simulink model "AngleSpeedToPWM"  (R2014a)
settings: Solver=FixedStepDiscrete  StartTime=0.0  StopTime=500000  FixedStep=1  RelTol=1e-3
libraries: hdlsllib x3
settings Model: Creator=sun.yifa  LastModifiedBy=rogers.a
settings OptimizationCC: BlockReduction=off  ConditionallyExecuteInputs=off  InlineParams=on
settings DebuggingCC: AlgebraicLoopMsg=error
settings HardwareCC: ProdHWDeviceType=ASIC/FPGA->ASIC/FPGA  ProdEqTarget=off

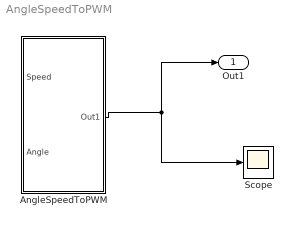
== system AngleSpeedToPWM ==
  "AngleSpeedToPWM " : Subsystem
  Scope : Scope
      settings: SaveName=ScopeData2
  Out1 : Outport  OutDataTypeStr=boolean
  wires:
  "AngleSpeedToPWM "/1(Out1) -> Scope/1, Out1/1

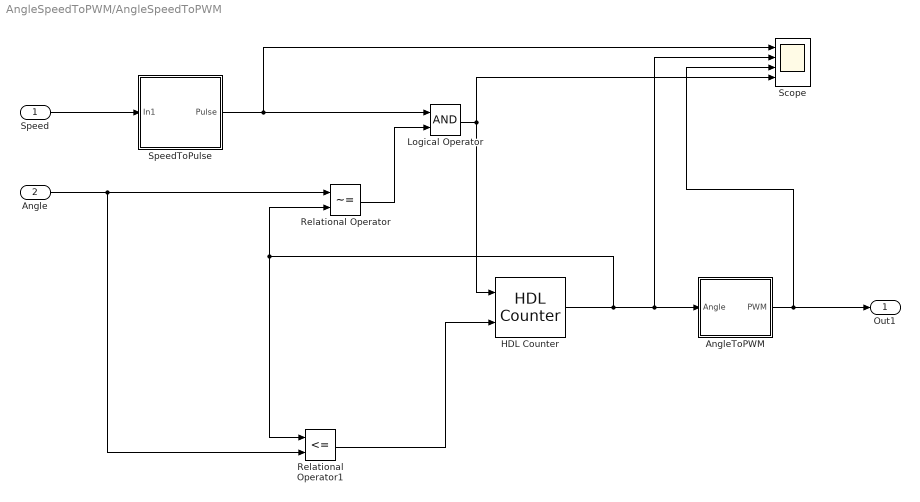
== system AngleSpeedToPWM/AngleSpeedToPWM  ==
  Speed : Inport
  Angle : Inport  Port=2
  "AngleToPWM " : Subsystem
  HDL Counter : hdlsllib/HDL Operations/HDL Counter  CountType=Count limited  CountInit=0  CountStep=1  CountMax=180  CountFromType=Specify  CountFrom=0  CountResetPort=off  CountLoadPort=off  CountEnbPort=on  CountDirPort=on  CountDataType=Unsigned  CountWordLen=8  CountFracLen=0  CountSampTime=1
  Logical Operator : Logic  AllPortsSameDT=off  OutDataTypeStr=boolean
  Relational Operator : RelationalOperator  Operator=~=  OutDataTypeStr=boolean
  Relational Operator1 : RelationalOperator  Operator=<=  OutDataTypeStr=boolean
  Scope : Scope  NumInputPorts=4
      settings: YMin=0~0~0~0  YMax=1~300~1~1
  SpeedToPulse : Subsystem
  Out1 : Outport  OutDataTypeStr=boolean
  wires:
  Speed/1 -> SpeedToPulse/1(In1)
  SpeedToPulse/1(Pulse) -> Logical Operator/1, Scope/1
  Angle/1 -> Relational Operator1/2, Relational Operator/1
  Relational Operator/1 -> Logical Operator/2
  Logical Operator/1 -> HDL Counter/1, Scope/4
  Relational Operator1/1 -> HDL Counter/2
  HDL Counter/1 -> Relational Operator/2, Relational Operator1/1, Scope/2, "AngleToPWM "/1("Angle ")
  "AngleToPWM "/1("PWM ") -> Out1/1, Scope/3

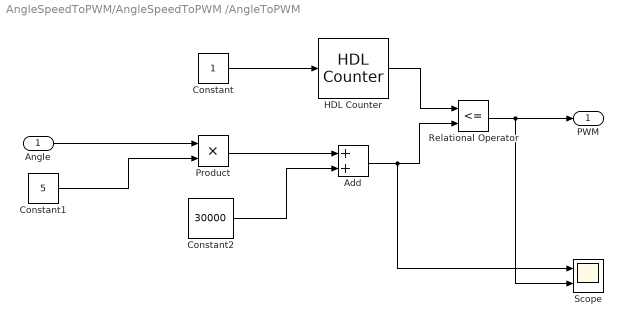
== system AngleSpeedToPWM/AngleSpeedToPWM /AngleToPWM  ==
  "Angle " : Inport  OutDataTypeStr=uint8
  Add : Sum
  Constant : Constant  OutDataTypeStr=boolean
  Constant1 : Constant  Value=5  OutDataTypeStr=uint32
  Constant2 : Constant  Value=30000  OutDataTypeStr=uint32
  HDL Counter : hdlsllib/HDL Operations/HDL Counter  CountType=Count limited  CountInit=0  CountStep=1  CountMax=10000  CountFromType=Initial value  CountFrom=0  CountResetPort=off  CountLoadPort=off  CountEnbPort=on  CountDirPort=off  CountDataType=Unsigned  CountWordLen=32  CountFracLen=0  CountSampTime=1
  Product : Product  OutDataTypeStr=Inherit: Inherit via back propagation  SaturateOnIntegerOverflow=on
  Relational Operator : RelationalOperator  Operator=<=  OutDataTypeStr=boolean
  Scope : Scope  NumInputPorts=2
      settings: YMin=45000~-5  YMax=45000~5
  "PWM " : Outport
  wires:
  HDL Counter/1 -> Relational Operator/1
  Constant2/1 -> Add/2
  Constant/1 -> HDL Counter/1
  Constant1/1 -> Product/2
  Product/1 -> Add/1
  "Angle "/1 -> Product/1
  Relational Operator/1 -> Scope/2, "PWM "/1
  Add/1 -> Scope/1, Relational Operator/2

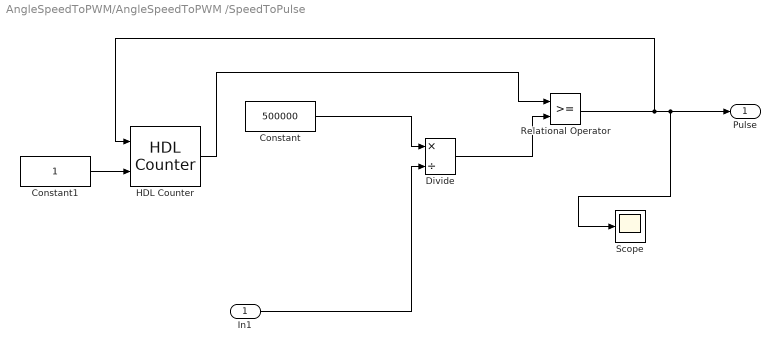
== system AngleSpeedToPWM/AngleSpeedToPWM /SpeedToPulse ==
  In1 : Inport
  Constant : Constant  Value=500000  OutDataTypeStr=int32
  Constant1 : Constant  OutDataTypeStr=boolean
  Divide : Product  Inputs=*/  SaturateOnIntegerOverflow=on  RndMeth=Zero
  HDL Counter : hdlsllib/HDL Operations/HDL Counter  CountType=Free running  CountInit=0  CountStep=1  CountMax=10000  CountFromType=Initial value  CountFrom=0  CountResetPort=on  CountLoadPort=off  CountEnbPort=on  CountDirPort=off  CountDataType=Unsigned  CountWordLen=32  CountFracLen=0  CountSampTime=1
  Relational Operator : RelationalOperator  OutDataTypeStr=boolean
  Scope : Scope
  Pulse : Outport
  wires:
  HDL Counter/1 -> Relational Operator/1
  Constant/1 -> Divide/1
  Divide/1 -> Relational Operator/2
  In1/1 -> Divide/2
  Relational Operator/1 -> Pulse/1, Scope/1, HDL Counter/1
  Constant1/1 -> HDL Counter/2
